simulink library "PCMULib"  (R2022b)
settings: Solver=ode45  StartTime=0.0  StopTime=10.0  RelTol=1e-3  EnableMultiTasking=on
undefined symbols (not defined in the file or in its folder): BreakpointData, BreakpointData1, BreakpointData2, BreakpointData_One_A, BreakpointData_Two_A, caaaa_dbi, caaaa_swi, cTmComprCtrl_n_i16SM4CmpHeatKiMax, cTmComprCtrl_n_i16SM4CmpHeatKiMin, cTmComprCtrl_n_i16SM4CmpHeatKpMax, cTmComprCtrl_n_i16SM4CmpHeatKpMin, cTmComprCtrl_Te_s32ErrCmpPIContinueHeatH, cTmComprCtrl_Te_s32ErrCmpPIContinueHeatL, cTmIn_n_ElacCmprReq_db, cTmIn_n_ElacCmprReq_sw, db, dbi, E2E_P01DataIDMode, E2E_P01ReceiverStatusType, EnumClass, iBit, initalValue, No_Runnable_Period, ObB_EidBsgStDerat_C, p_OVERRIDE_MASTER_SWITCH, SlDemoSign, sw, swi, SwitchOff_P, SwitchOn_P, Table, TableData_M, VCCTi33, VSysD_FidVehDerat1_C
libraries: simulink x22, CCMLib x11, simulink_need_slupdate x9, UXFD_Lib x7, canmsglib x2, PTCC_Lib x1, hdlsllib x1
(part 3 of 7)

== system PCMULib/CCM/Rate Limiter Resettable IC ==
  up : Inport  OutDataTypeStr=InputOutputDataType
  u : Inport  Port=2  OutDataTypeStr=InputOutputDataType
  IC : Inport  Port=3  OutDataTypeStr=InputOutputDataType
  T : Inport  Port=4  OutDataTypeStr=VCCTiSamplePerd
  lo : Inport  Port=5  OutDataTypeStr=InputOutputDataType
  R : Inport  Port=6  OutDataTypeStr=boolean
  Data Type Conversion{1..5} (5 alike) : DataTypeConversion  OutDataTypeStr=single  RndMeth=Floor
  Difference Inputs1 : Sum  Description=Add in CPU  DisableCoverage=on  Inputs=+-  OutDataTypeStr=single  SaturateOnIntegerOverflow=on
  Difference Inputs2 : Sum  Description=Add in CPU  OutDataTypeStr=single  SaturateOnIntegerOverflow=on
  FixPt Data Type Duplicate : DataTypeDuplicate  DisableCoverage=on  NumInputPorts=7
  Saturation Dynamic : simulink/Discontinuities/Saturation Dynamic  OutMin=[]  OutMax=[]  OutDataTypeStr=single  OutputDataTypeScalingMode=single  OutDataType=dataType  OutScaling=[]  DoSatur=on
  Switch : Switch  Criteria=u2 ~= 0  InputSameDT=off
  Unit Delay Resettable External IC boolean controlled : Subsystem  mask(Unit Delay Resettable External Initial Condition (boolean)){dt=single, UnitDelayInitCondition=0}
      mask prompts: dt "Data type in/out"; UnitDelayInitCondition "Internal unit delay block initial condition:"
      mask help:
      | This is the same block as the Simulink standard, except all fix point
      | data-types have been changed to booleans.
      | The internal unit delay block can often be kept as 0, unless the input/output signal is of ENUM type.
      | Made by Niklas Magnusson (nmagnus3).
      | NGCC
      mask Display: dpoly(1,[1 0],'z')
  dataType : DataTypeConversion  OutDataTypeStr=InputOutputDataType  RndMeth=Floor
  delta fall limit : Product  DisableCoverage=on  Inputs=**  OutDataTypeStr=single  SaturateOnIntegerOverflow=on
  delta rise limit : Product  DisableCoverage=on  Inputs=**  OutDataTypeStr=single  SaturateOnIntegerOverflow=on
  Y : Outport  OutDataTypeStr=InputOutputDataType  InitialOutput=0
  wires:
  Switch/1 -> dataType/1
  Data Type Conversion5/1 -> delta rise limit/2, delta fall limit/1
  R/1 -> Switch/2, Unit Delay Resettable External IC boolean controlled/2(R)
  IC/1 -> Data Type Conversion3/1
  Difference Inputs1/1 -> FixPt Data Type Duplicate/4, Saturation Dynamic/2
  u/1 -> Data Type Conversion2/1
  delta fall limit/1 -> FixPt Data Type Duplicate/3, Saturation Dynamic/3
  Saturation Dynamic/1 -> Difference Inputs2/1, FixPt Data Type Duplicate/7
  Unit Delay Resettable External IC boolean controlled/1(y) -> Difference Inputs2/2, Difference Inputs1/2, FixPt Data Type Duplicate/2
  Difference Inputs2/1 -> Switch/3, FixPt Data Type Duplicate/1, Unit Delay Resettable External IC boolean controlled/1(u)
  up/1 -> Data Type Conversion1/1
  delta rise limit/1 -> FixPt Data Type Duplicate/6, Saturation Dynamic/1
  lo/1 -> Data Type Conversion4/1
  T/1 -> Data Type Conversion5/1
  Data Type Conversion1/1 -> delta rise limit/1
  Data Type Conversion2/1 -> Difference Inputs1/1, FixPt Data Type Duplicate/5
  Data Type Conversion3/1 -> Switch/1, Unit Delay Resettable External IC boolean controlled/3(IC)
  Data Type Conversion4/1 -> delta fall limit/2
  dataType/1 -> Y/1

== system PCMULib/CCM/SR_latch ==
  Set : Inport  OutDataTypeStr=boolean
  Reset : Inport  Port=2  OutDataTypeStr=boolean
  Logical Operator : Logic  AllPortsSameDT=off  OutDataTypeStr=boolean
  Logical Operator1 : Logic  Operator=OR  AllPortsSameDT=off  OutDataTypeStr=boolean
  Logical Operator2 : Logic  Operator=NOT  AllPortsSameDT=off  OutDataTypeStr=boolean
  Unit Delay External IC : simulink_need_slupdate/Unit Delay External IC  tsamp=-1
  false : Constant  Value=false  OutDataTypeStr=boolean  SampleTime=-1
  SetState : Outport  OutDataTypeStr=boolean
  wires:
  Set/1 -> Logical Operator1/2
  false/1 -> Unit Delay External IC/2
  Unit Delay External IC/1 -> Logical Operator1/1
  Logical Operator2/1 -> Logical Operator/2
  Reset/1 -> Logical Operator2/1
  Logical Operator1/1 -> Logical Operator/1
  Logical Operator/1 -> Unit Delay External IC/1, SetState/1

== system PCMULib/CCM/SR_latch_NoRst ==
  Set : Inport  OutDataTypeStr=boolean
  Logical Operator1 : Logic  Operator=OR  AllPortsSameDT=off  OutDataTypeStr=boolean
  Unit Delay External IC : simulink_need_slupdate/Unit Delay External IC  tsamp=-1
  false : Constant  Value=false  OutDataTypeStr=boolean  SampleTime=-1
  SetState : Outport  OutDataTypeStr=boolean
  wires:
  Logical Operator1/1 -> SetState/1, Unit Delay External IC/1
  Unit Delay External IC/1 -> Logical Operator1/1
  false/1 -> Unit Delay External IC/2
  Set/1 -> Logical Operator1/2

== system PCMULib/CCM/Timer ==
  note: CounterRunning
  note: If timer is set to zero, use start/hold/reset-status as output.
      | This is to avoid TimerFinished to be set to true without even the timer has started.
  Start : Inport  OutDataTypeStr=boolean
  Reset : Inport  Port=2  OutDataTypeStr=boolean
  Time : Inport  Port=3  OutDataTypeStr=timeDataType
  Divide : Product  Inputs=*/  OutDataTypeStr=VCCUInt32  RndMeth=Round  SaturateOnIntegerOverflow=on
  IC : Constant  Value=0  OutDataTypeStr=VCCUInt32  SampleTime=-1
  Increment : Constant  OutDataTypeStr=VCCUInt32  SampleTime=-1
  Logical Operator : Logic  AllPortsSameDT=off  OutDataTypeStr=boolean
  Logical Operator2 : Logic  Operator=OR  AllPortsSameDT=off  OutDataTypeStr=boolean
  Logical Operator3 : Logic  Operator=NOT  AllPortsSameDT=off  OutDataTypeStr=boolean
  Relational Operator : RelationalOperator  OutDataTypeStr=boolean  InputSameDT=off
  Relational Operator1 : RelationalOperator  Operator=>  OutDataTypeStr=boolean  InputSameDT=off
  RunnablePeriod : Constant  Value=RunnablePeriod  OutDataTypeStr=VCCTiSamplePerd  SampleTime=-1
  StopCounter : Constant  Value=0  OutDataTypeStr=VCCUInt32  SampleTime=-1
  Sum : Sum  OutDataTypeStr=VCCUInt32  SaturateOnIntegerOverflow=on
  Switch : Switch  Criteria=u2 ~= 0  InputSameDT=off
  Switch1 : Switch  Criteria=u2 ~= 0  InputSameDT=off
  Unit Delay External IC : simulink_need_slupdate/Unit Delay External IC  tsamp=-1
  Unit Delay Resettable External IC1 : CCMLib/Unit Delay Resettable External IC  dataType=VCCUInt32
  ZeroTicks : Constant  Value=0  OutDataTypeStr=VCCUInt32  SampleTime=-1
  false : Constant  Value=false  OutDataTypeStr=boolean  SampleTime=-1
  TimerFinished : Outport  OutDataTypeStr=boolean
  wires:
  Logical Operator2/1 -> Logical Operator/1
  false/1 -> Unit Delay External IC/2
  Logical Operator/1 -> Switch/2, Unit Delay External IC/1, Switch1/3
  Start/1 -> Logical Operator2/2
  Unit Delay External IC/1 -> Logical Operator2/1
  Unit Delay Resettable External IC1/1 -> Sum/1, Relational Operator/1
  Switch/1 -> Sum/2
  Increment/1 -> Switch/1
  StopCounter/1 -> Switch/3
  RunnablePeriod/1 -> Divide/2
  ZeroTicks/1 -> Relational Operator1/2
  Relational Operator1/1 -> Switch1/2
  Relational Operator/1 -> Switch1/1
  Divide/1 -> Relational Operator/2, Relational Operator1/1
  Switch1/1 -> TimerFinished/1
  Logical Operator3/1 -> Logical Operator/2
  Reset/1 -> Logical Operator3/1, Unit Delay Resettable External IC1/3
  Time/1 -> Divide/1
  IC/1 -> Unit Delay Resettable External IC1/2
  Sum/1 -> Unit Delay Resettable External IC1/1

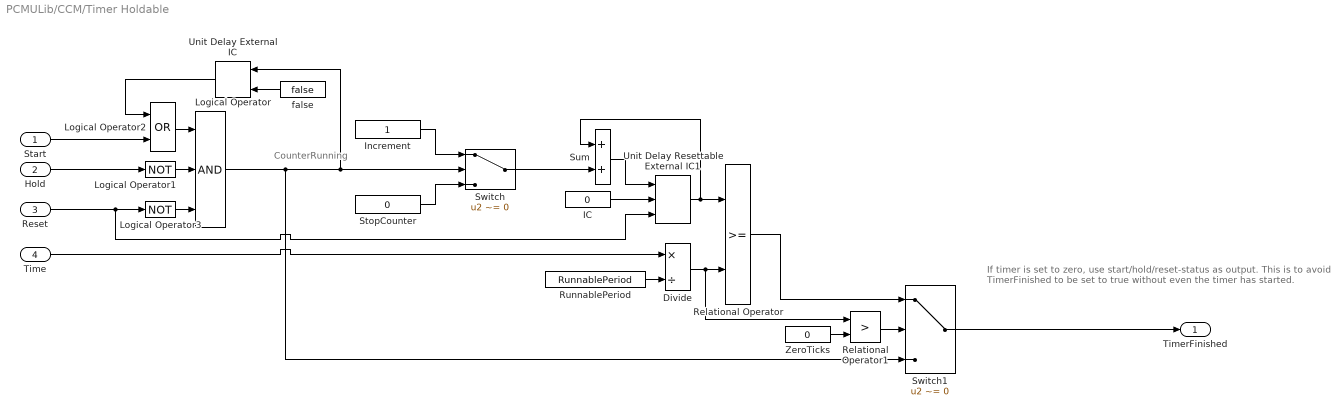
== system PCMULib/CCM/Timer Holdable ==
  note: If timer is set to zero, use start/hold/reset-status as output.
      | This is to avoid TimerFinished to be set to true without even the timer has started.
  note: CounterRunning
  Start : Inport  OutDataTypeStr=boolean
  Hold : Inport  Port=2  OutDataTypeStr=boolean
  Reset : Inport  Port=3  OutDataTypeStr=boolean
  Time : Inport  Port=4  OutDataTypeStr=timeDataType
  Divide : Product  Inputs=*/  OutDataTypeStr=VCCUInt32  RndMeth=Round  SaturateOnIntegerOverflow=on
  IC : Constant  Value=0  OutDataTypeStr=VCCUInt32  SampleTime=-1
  Increment : Constant  OutDataTypeStr=VCCUInt32  SampleTime=-1
  Logical Operator : Logic  Inputs=3  AllPortsSameDT=off  OutDataTypeStr=boolean
  Logical Operator1 : Logic  Operator=NOT  AllPortsSameDT=off  OutDataTypeStr=boolean
  Logical Operator2 : Logic  Operator=OR  AllPortsSameDT=off  OutDataTypeStr=boolean
  Logical Operator3 : Logic  Operator=NOT  AllPortsSameDT=off  OutDataTypeStr=boolean
  Relational Operator : RelationalOperator  OutDataTypeStr=boolean  InputSameDT=off
  Relational Operator1 : RelationalOperator  Operator=>  OutDataTypeStr=boolean  InputSameDT=off
  RunnablePeriod : Constant  Value=RunnablePeriod  OutDataTypeStr=VCCTiSamplePerd  SampleTime=-1
  StopCounter : Constant  Value=0  OutDataTypeStr=VCCUInt32  SampleTime=-1
  Sum : Sum  OutDataTypeStr=VCCUInt32  SaturateOnIntegerOverflow=on
  Switch : Switch  Criteria=u2 ~= 0  InputSameDT=off
  Switch1 : Switch  Criteria=u2 ~= 0  InputSameDT=off
  Unit Delay External IC : simulink_need_slupdate/Unit Delay External IC  tsamp=-1
  Unit Delay Resettable External IC1 : CCMLib/Unit Delay Resettable External IC  dataType=VCCUInt32
  ZeroTicks : Constant  Value=0  OutDataTypeStr=VCCUInt32  SampleTime=-1
  false : Constant  Value=false  OutDataTypeStr=boolean  SampleTime=-1
  TimerFinished : Outport  OutDataTypeStr=boolean
  wires:
  Sum/1 -> Unit Delay Resettable External IC1/1
  IC/1 -> Unit Delay Resettable External IC1/2
  Time/1 -> Divide/1
  Reset/1 -> Unit Delay Resettable External IC1/3, Logical Operator3/1
  Logical Operator3/1 -> Logical Operator/3
  Switch1/1 -> TimerFinished/1
  Divide/1 -> Relational Operator1/1, Relational Operator/2
  Relational Operator/1 -> Switch1/1
  Relational Operator1/1 -> Switch1/2
  ZeroTicks/1 -> Relational Operator1/2
  RunnablePeriod/1 -> Divide/2
  StopCounter/1 -> Switch/3
  Increment/1 -> Switch/1
  Switch/1 -> Sum/2
  Unit Delay Resettable External IC1/1 -> Relational Operator/1, Sum/1
  Unit Delay External IC/1 -> Logical Operator2/1
  Start/1 -> Logical Operator2/2
  Logical Operator/1 -> Switch1/3, Unit Delay External IC/1, Switch/2
  false/1 -> Unit Delay External IC/2
  Logical Operator2/1 -> Logical Operator/1
  Hold/1 -> Logical Operator1/1
  Logical Operator1/1 -> Logical Operator/2

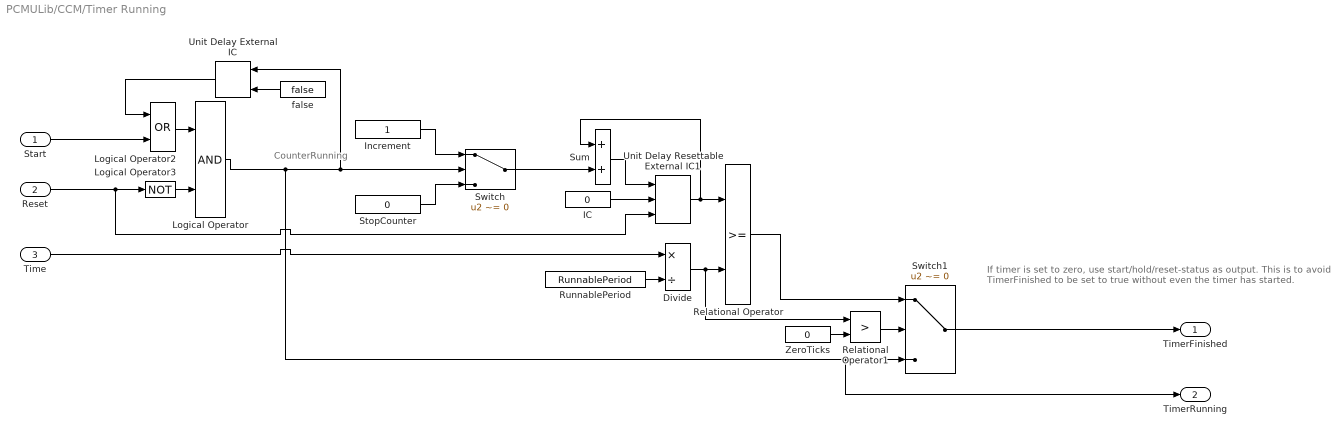
== system PCMULib/CCM/Timer Running ==
  note: If timer is set to zero, use start/hold/reset-status as output.
      | This is to avoid TimerFinished to be set to true without even the timer has started.
  note: CounterRunning
  Start : Inport  OutDataTypeStr=boolean
  Reset : Inport  Port=2  OutDataTypeStr=boolean
  Time : Inport  Port=3  OutDataTypeStr=timeDataType
  Divide : Product  Inputs=*/  OutDataTypeStr=VCCUInt32  RndMeth=Round  SaturateOnIntegerOverflow=on
  IC : Constant  Value=0  OutDataTypeStr=VCCUInt32  SampleTime=-1
  Increment : Constant  OutDataTypeStr=VCCUInt32  SampleTime=-1
  Logical Operator : Logic  AllPortsSameDT=off  OutDataTypeStr=boolean
  Logical Operator2 : Logic  Operator=OR  AllPortsSameDT=off  OutDataTypeStr=boolean
  Logical Operator3 : Logic  Operator=NOT  AllPortsSameDT=off  OutDataTypeStr=boolean
  Relational Operator : RelationalOperator  OutDataTypeStr=boolean  InputSameDT=off
  Relational Operator1 : RelationalOperator  Operator=>  OutDataTypeStr=boolean  InputSameDT=off
  RunnablePeriod : Constant  Value=RunnablePeriod  OutDataTypeStr=VCCTiSamplePerd  SampleTime=-1
  StopCounter : Constant  Value=0  OutDataTypeStr=VCCUInt32  SampleTime=-1
  Sum : Sum  OutDataTypeStr=VCCUInt32  SaturateOnIntegerOverflow=on
  Switch : Switch  Criteria=u2 ~= 0  InputSameDT=off
  Switch1 : Switch  Criteria=u2 ~= 0  InputSameDT=off
  Unit Delay External IC : simulink_need_slupdate/Unit Delay External IC  tsamp=-1
  Unit Delay Resettable External IC1 : CCMLib/Unit Delay Resettable External IC  dataType=VCCUInt32
  ZeroTicks : Constant  Value=0  OutDataTypeStr=VCCUInt32  SampleTime=-1
  false : Constant  Value=false  OutDataTypeStr=boolean  SampleTime=-1
  TimerFinished : Outport  OutDataTypeStr=boolean
  TimerRunning : Outport  Port=2  OutDataTypeStr=boolean
  wires:
  Sum/1 -> Unit Delay Resettable External IC1/1
  IC/1 -> Unit Delay Resettable External IC1/2
  Time/1 -> Divide/1
  Reset/1 -> Unit Delay Resettable External IC1/3, Logical Operator3/1
  Logical Operator3/1 -> Logical Operator/2
  Switch1/1 -> TimerFinished/1
  Divide/1 -> Relational Operator1/1, Relational Operator/2
  Relational Operator/1 -> Switch1/1
  Relational Operator1/1 -> Switch1/2
  ZeroTicks/1 -> Relational Operator1/2
  RunnablePeriod/1 -> Divide/2
  StopCounter/1 -> Switch/3
  Increment/1 -> Switch/1
  Switch/1 -> Sum/2
  Unit Delay Resettable External IC1/1 -> Sum/1, Relational Operator/1
  Unit Delay External IC/1 -> Logical Operator2/1
  Start/1 -> Logical Operator2/2
  Logical Operator/1 -> TimerRunning/1, Switch1/3, Unit Delay External IC/1, Switch/2
  false/1 -> Unit Delay External IC/2
  Logical Operator2/1 -> Logical Operator/1

== system PCMULib/CCM/Unit Delay External IC ==
  u : Inport  OutDataTypeStr=dataType
  IC : Inport  Port=2  OutDataTypeStr=dataType
  Constant : Constant  Value=true  OutDataTypeStr=boolean  SampleTime=-1
  Switch : Switch  Criteria=u2 ~= 0  InputSameDT=off
  Unit Delay : UnitDelay  InitialCondition=false  SampleTime=-1  HasFrameUpgradeWarning=on
      settings: AttributesFormatString=X0=%<X0>
  Unit Delay1 : UnitDelay  SampleTime=-1  HasFrameUpgradeWarning=on
      settings: AttributesFormatString=X0=%<X0>
  y : Outport  OutDataTypeStr=dataType
  wires:
  Switch/1 -> y/1
  IC/1 -> Switch/3
  u/1 -> Unit Delay1/1
  Unit Delay1/1 -> Switch/1
  Constant/1 -> Unit Delay/1
  Unit Delay/1 -> Switch/2

== system PCMULib/CCM/Unit Delay Resettable ==
  u : Inport  OutDataTypeStr=dataType
  R : Inport  Port=2  OutDataTypeStr=boolean
  Constant : Constant  Value=false  OutDataTypeStr=boolean  SampleTime=-1
  Logical Operator : Logic  Operator=OR  AllPortsSameDT=off  OutDataTypeStr=boolean
  Logical Operator1 : Logic  Operator=NOT  AllPortsSameDT=off  OutDataTypeStr=boolean
  Switch : Switch  Criteria=u2 ~= 0  InputSameDT=off
  Switch1 : Switch  Criteria=u2 ~= 0  InputSameDT=off
  Unit Delay : UnitDelay  InitialCondition=true  SampleTime=-1  HasFrameUpgradeWarning=on
      settings: AttributesFormatString=X0=%<X0>
  Unit Delay1 : UnitDelay  InitialCondition=initialCondition  SampleTime=-1  HasFrameUpgradeWarning=on
      settings: AttributesFormatString=X0=%<X0>
  initialCondition : Constant  Value=initialCondition  OutDataTypeStr=dataType  SampleTime=-1
  y : Outport  OutDataTypeStr=dataType
  wires:
  Constant/1 -> Unit Delay/1
  Switch/1 -> y/1
  Logical Operator/1 -> Switch/2
  Unit Delay/1 -> Logical Operator/2
  R/1 -> Logical Operator/1, Logical Operator1/1
  Logical Operator1/1 -> Switch1/2
  initialCondition/1 -> Switch1/3, Switch/1
  Switch1/1 -> Unit Delay1/1
  Unit Delay1/1 -> Switch/3
  u/1 -> Switch1/1

== system PCMULib/CCM/Unit Delay Resettable External IC ==
  u : Inport  OutDataTypeStr=dataType
  IC : Inport  Port=2  OutDataTypeStr=dataType
  R : Inport  Port=3  OutDataTypeStr=boolean
  Constant : Constant  Value=true  OutDataTypeStr=boolean  SampleTime=-1
  Logical Operator : Logic  Operator=NOT  AllPortsSameDT=off  OutDataTypeStr=boolean
  Logical Operator1 : Logic  AllPortsSameDT=off  OutDataTypeStr=boolean
  Switch : Switch  Criteria=u2 ~= 0  InputSameDT=off
  Switch1 : Switch  Criteria=u2 ~= 0  InputSameDT=off
  Unit Delay : UnitDelay  InitialCondition=false  SampleTime=-1  HasFrameUpgradeWarning=on
      settings: AttributesFormatString=X0=%<X0>
  Unit Delay1 : UnitDelay  SampleTime=-1  HasFrameUpgradeWarning=on
      settings: AttributesFormatString=X0=%<X0>
  y : Outport  OutDataTypeStr=dataType
  wires:
  Logical Operator1/1 -> Switch/2
  Unit Delay/1 -> Logical Operator1/1
  Switch1/1 -> Unit Delay1/1
  IC/1 -> Switch/3, Switch1/3
  u/1 -> Switch1/1
  R/1 -> Logical Operator/1
  Logical Operator/1 -> Logical Operator1/2, Switch1/2
  Constant/1 -> Unit Delay/1
  Unit Delay1/1 -> Switch/1
  Switch/1 -> y/1

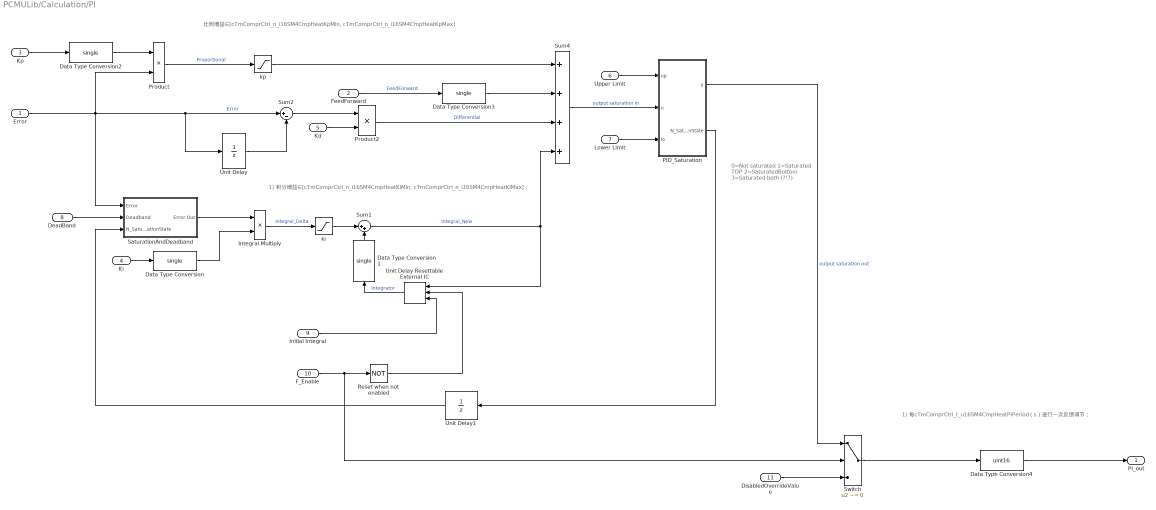
== system PCMULib/Calculation/PI ==
  note: 1) 积分增益∈[cTmComprCtrl_n_i16SM4CmpHeatKiMin, cTmComprCtrl_n_i16SM4CmpHeatKiMax]；
  note: 比例增益∈[cTmComprCtrl_n_i16SM4CmpHeatKpMin, cTmComprCtrl_n_i16SM4CmpHeatKpMax]
  note: 1) 每cTmComprCtrl_t_u16SM4CmpHeatPIPeriod（s）进行一次反馈调节；
  note: 0=Not saturated
      | 1=Saturated TOP
      | 2=SaturatedBottom
      | 3=Saturated both (?!?)
  Error : Inport  OutDataTypeStr=single
  FeedForward : Inport  Port=2  OutDataTypeStr=uint16
  Kp : Inport  Port=3  OutDataTypeStr=uint16
  Ki : Inport  Port=4  OutDataTypeStr=uint16
  Kd : Inport  Port=5  OutDataTypeStr=single
  Upper Limit : Inport  Port=6  OutDataTypeStr=single
  Lower Limit : Inport  Port=7  OutDataTypeStr=single
  DeadBand : Inport  Port=8  OutDataTypeStr=single
  Initial Integral : Inport  Port=9  OutDataTypeStr=single
  F_Enable : Inport  Port=10  OutDataTypeStr=boolean
  DisabledOverrideValue : Inport  Port=11  OutDataTypeStr=single
  Data Type Conversion{,1..3} (4 alike) : DataTypeConversion  OutDataTypeStr=single  SaturateOnIntegerOverflow=off  RndMeth=Floor
  Data Type Conversion4 : DataTypeConversion  OutDataTypeStr=uint16  SaturateOnIntegerOverflow=off  RndMeth=Floor
  Integral Multiply : Product  OutDataTypeStr=single  RndMeth=Zero  SaturateOnIntegerOverflow=on
  PID_Saturation : Subsystem  mask(Saturation Dynamic){OutMin=[], OutMax=[], OutDataTypeStr=Inherit: Same as second input, OutputDataTypeScalingMode=Same as second input, OutDataType=FloatBit1, OutScaling=[], LockScale=off, RndMeth=Nearest, DoSatur=on}
      mask prompts: OutMin "Output minimum:"; OutMax "Output maximum:"; OutDataTypeStr "Output data type:"; OutputDataTypeScalingMode "Output data type mode:"; OutDataType "Output data type (e.g. fixdt(1, 16), fixdt('single')):"; OutScaling "Output scaling (Slope, e.g. 2^-9 or [Slope Bias], e.g. [1.25 3]):"; LockScale "Lock output data type setting against changes by the fixed-point tools"; RndMeth "Integer rounding mode:"; DoSatur "Saturate on integer overflow"
      mask help: Bound the range of the second input by using the first input (upper limit) and the third input (lower limit).
      mask init:
      | blkH = gcbh;
      | blkName = getfullname(blkH);
      | 
      | switch_blks = {'Switch','Switch2'}; 
      | for i = 1:length(switch_blks)
      |   set_param([blkName,'/',switch_blks{i}], ...
      |       'RndMeth', RndMeth, ...
      | 	  'DoSatur', DoSatur);
      | end
      | 
      | propBlk = [blkName, '/Data Type Propagation'];
      | 
      | if strcmp(OutputDataTypeScalingMode, 'Same as second input')
      |     set_param(propBlk, 'PropDataTypeMode', 'Inherit via propagation rule', ...
      |                        'PropScalingMode',  'Inherit via propagation rule');
      | else
      |     scaling = OutScaling;
      |     switch OutputDataTypeScalingMode
      |       case 'double'
      |         dataType = 'fixdt(''double'')';
      |       case 'single'
      |         dataType = 'fixdt(''single'')';
      |       case 'int8'
      |         dataType = 'fixdt(1,8,0)';
      |       case 'uint8'
      |         dataType = 'fixdt(0,8,0)';
      |       case 'int16'
      |         dataType = 'fixdt(1,16,0)';
      |       case 'uint16'
      |         dataType = 'fixdt(0,16,0)';
      |       case 'int32'
      |         dataType = 'fixdt(1,32,0)';
      |       case 'uint32'
      |         dataType = 'fixdt(0,32,0)';
      |       case 'Specify via dialog'
      |         dataType = OutDataType;
      |     end
      |     
      |     set_param(propBlk, 'PropDataTypeMode', 'Specify via dialog', ...
      |                        'PropScalingMode',  'Specify via dialog', ...
      |                        'PropDataType',     dataType, ...
      |                        'PropScaling',      scaling);
      | end
      mask Callback OutDataTypeStr: fixptdialog(gcbh)
      mask TypeOptions OutputDataTypeScalingMode: double | single | int8 | uint8 | int16 | uint16 | int32 | uint32 | Specify via dialog | Same as second input
      mask Callback OutputDataTypeScalingMode: fixptdialog(gcbh)
      mask Callback OutDataType: fixptdialog(gcbh)
      mask TypeOptions RndMeth: Ceiling | Convergent | Floor | Nearest | Round | Simplest | Zero
      mask Display: plot([0.15 0.85],[.5 .5],[.5 .5],[0.05 0.95],0.15+0.7*[0 .25 .75 1],0.05+0.9*[.25 .25 .75 .75]);
  Product : Product  OutDataTypeStr=single  RndMeth=Zero
  Product2 : Product  OutDataTypeStr=single  RndMeth=Zero  SaturateOnIntegerOverflow=on
  Reset when not enabled : Logic  Operator=NOT  Inputs=1  AllPortsSameDT=off  OutDataTypeStr=boolean
  SaturationAndDeadband : Subsystem
  Sum1 : Sum  Inputs=|++  InputSameDT=on  AccumDataTypeStr=single  OutDataTypeStr=single  SaturateOnIntegerOverflow=on
  Sum2 : Sum  Inputs=|+-  SaturateOnIntegerOverflow=on
  Sum4 : Sum  Inputs=++++  RndMeth=Nearest  SaturateOnIntegerOverflow=on
  Switch : Switch  Criteria=u2 ~= 0  SaturateOnIntegerOverflow=off  InputSameDT=off
  Unit Delay : UnitDelay  SampleTime=-1  HasFrameUpgradeWarning=on
  Unit Delay Resettable External IC : simulink_need_slupdate/Unit Delay Resettable External IC  tsamp=-1
  Unit Delay1 : UnitDelay  SampleTime=-1  HasFrameUpgradeWarning=on
  ki : Saturate  UpperLimit=cTmComprCtrl_n_i16SM4CmpHeatKiMax  LowerLimit=cTmComprCtrl_n_i16SM4CmpHeatKiMin
  kp : Saturate  UpperLimit=cTmComprCtrl_n_i16SM4CmpHeatKpMax  LowerLimit=cTmComprCtrl_n_i16SM4CmpHeatKpMin
  PI_out : Outport  OutDataTypeStr=uint16  VectorParamsAs1DForOutWhenUnconnected=off
  wires:
  Product2/1 -> Sum4/3  "Differential"
  Sum1/1 -> Sum4/4, Unit Delay Resettable External IC/1  "Integral_New"
  Upper Limit/1 -> PID_Saturation/1(up)
  DeadBand/1 -> SaturationAndDeadband/2(Deadband)
  Unit Delay/1 -> Sum2/2
  Kd/1 -> Product2/2
  DisabledOverrideValue/1 -> Switch/3
  Error/1 -> SaturationAndDeadband/1(Error), Product/2, Sum2/1, Unit Delay/1  "Error"
  Sum2/1 -> Product2/1
  Unit Delay Resettable External IC/1 -> Data Type Conversion1/1  "Integrator"
  Kp/1 -> Data Type Conversion2/1
  PID_Saturation/1(y) -> Switch/1  "output saturation out"
  Reset when not enabled/1 -> Unit Delay Resettable External IC/2
  Initial Integral/1 -> Unit Delay Resettable External IC/3
  Lower Limit/1 -> PID_Saturation/3(lo)
  SaturationAndDeadband/1(Error Out) -> Integral Multiply/1
  Sum4/1 -> PID_Saturation/2(u)  "output saturation in"
  FeedForward/1 -> Data Type Conversion3/1  "FeedForward"
  F_Enable/1 -> Reset when not enabled/1, Switch/2
  Unit Delay1/1 -> SaturationAndDeadband/3(N_SaturationState)
  Product/1 -> kp/1  "Proportional"
  Integral Multiply/1 -> ki/1  "Integral_Delta"
  PID_Saturation/2(N_SaturationState) -> Unit Delay1/1
  Ki/1 -> Data Type Conversion/1
  Data Type Conversion1/1 -> Sum1/2
  kp/1 -> Sum4/1
  ki/1 -> Sum1/1
  Switch/1 -> Data Type Conversion4/1
  Data Type Conversion/1 -> Integral Multiply/2
  Data Type Conversion2/1 -> Product/1
  Data Type Conversion3/1 -> Sum4/2
  Data Type Conversion4/1 -> PI_out/1

== system PCMULib/Calculation/interpolation ==
  note: 外循环比例
  note: 内循环比例
  rate : Inport
  internal : Inport  Port=2
  external : Inport  Port=3
  Add1 : Sum  Inputs=-+
  Add2 : Sum
  Constant4 : Constant  OutDataTypeStr=single
  Constant5 : Constant  Value=100  OutDataTypeStr=single
  Data Type Conversion : DataTypeConversion  OutDataTypeStr=uint16  SaturateOnIntegerOverflow=off  RndMeth=Floor
  Product : Product
  Product1 : Product
  Product2 : Product  Inputs=*/
  rst : Outport
  wires:
  external/1 -> Product1/2
  Product1/1 -> Add2/2
  Add2/1 -> Data Type Conversion/1
  rate/1 -> Product2/1
  Constant4/1 -> Add1/2
  Product/1 -> Add2/1
  internal/1 -> Product/1
  Add1/1 -> Product1/1
  Constant5/1 -> Product2/2
  Product2/1 -> Product/2, Add1/1
  Data Type Conversion/1 -> rst/1

== system PCMULib/Custom/CAN ==
  note: CAN
  CAN Pack : canmsglib/CAN Pack  MsgList=(none)  MsgName=CAN Msg  MsgIDType=Standard (11-bit identifier)  MsgIdentifier=0  MsgLength=8  Remote=off  ApplyMinMax=off  BusOutput=off  SignalInfo={}
      settings: DataFormat=raw data
  CAN Unpack : canmsglib/CAN Unpack  MsgList=(none)  MsgName=CAN Msg  MsgIDType=Standard (11-bit identifier)  MsgIdentifier=0  MsgLength=8  SignalInfo={}  IDPort=off  TimestampPort=off  ErrorPort=off  RemotePort=off  LengthPort=off  StatusPort=off  ApplyMinMax=off
      settings: DataFormat=raw data
  CAN_Receive : Subsystem  mask(CAN Message Receive( GLib TM )){}
      mask help:
      | Input： DataType CAN_Message Signal and handle
      | Output：If Received success , Return Value is 1
      mask Display:
      | port_label('input',1,'Message')
      | port_label('input',2,'Handle')
      | port_label('output',1,'ReturnValue')
      | disp('ACTION_CANBSW_RecMsg_S')
  CAN_Transmit : Subsystem  mask(CAN Message Transmit( GLib TM )){}
      mask help:
      | Input： DataType CAN_Message Signal and handle
      | Output：If Transmited success , Return Value is 1
      mask Display:
      | port_label('input',1,'Message')
      | port_label('input',2,'Handle')
      | port_label('output',1,'ReturnValue')
      | disp('ACTION_CANBSW_SndMsg_S')
  CanHex2Signed : Subsystem  mask(CAN signal Hex2Signed){BitLengthValue=32, FactorValue=0.001, OffsetValue=0}
      mask prompts: BitLengthValue "CAN Signal Bit Length（0<u<=32bit）"; FactorValue "Factor"; OffsetValue "Offset"
      mask help: convert the hex to signed value, please specified bit length of varible in CAN matrix, the maximum bit length in CAN matrixa may be 32bit; Also, please specified the factor and offset, then execute Phy=hex*factor+offset.
      mask init:
      | % The mask parameter returns the one-based index of the selection
      | FactorValue;
      | OffsetValue;
      | BitLengthValue;
      | % To obtain the string corresponding to the selection, use get_param
      | blk = gcb;
      | FactorString = get_param(blk,'FactorValue');
      | OffsetString = get_param(blk,'OffsetValue');
      | BitSzieString = get_param(blk,'BitLengthValue');
      | 
      |     % Convert the string into a single to use the value under the mask
      |     BitLength = single(str2num(BitSzieString)); 
      |     Factor=single(str2num(FactorString)); 
      |     Offset=single(str2num(OffsetString));
      mask Display:
      | fprintf('CAN signal convert\nBitLength: %d\nFactor: %2.4f\nOffset: %2.4f',...
      |     BitLengthValue,FactorValue,OffsetValue);
  Get_MsgLength : Subsystem  mask(Get CAN Message Length( GLib TM )){}
      mask help:
      | Input： DataType CAN_Message Signal
      | Output：CAN Message Length
      mask Display:
      | port_label('input',1,'Message')
      | port_label('output',1,'Length')
      | disp('Msg_Length_S')
  xbackground1 : Subsystem
      mask Display: disp(' ')

== system PCMULib/Custom/Diagnose ==
  note: Diagnose
  Dem_SetEventStatus : Subsystem  mask(SL Blockset Dem_SetEventStatus){EventID=ObB_EidBsgStDerat_C}
      mask prompts: EventID "Dem Event ID"
      mask help:
      | Interface block to call Dem_SetEventStatus.
      | The output of the block can be captured by using Dem_SetEventStatus blocks with the same EventID.
      mask TypeOptions EventID: DEM_EventID/Value
      mask Display:
      | id = get_param(gcb,'EventID');
      | text(0.55,0.9,sprintf('Dem_SetEventStatus\nEventID: %s', id),...
      |     'horizontalAlignment','center',...
      |     'verticalAlignment', 'top');
      | 
      | 
      | port_label('input',1,'EveSt');
      | port_label('input',2,'bEna');
  Fim_GetFunctionPermission : Subsystem  mask(SL Blockset Fim_GetFunctionPermission){FunctionID=VSysD_FidVehDerat1_C}
      mask prompts: FunctionID "FIM FunctionID"
      mask help:
      | Interface block to call Fim_GetFunctionPermission.
      | The output of the block can be stimulated by using Fim_GetFunctionPermission_Stimuli blocks with the same FunctionID.
      mask TypeOptions FunctionID: FIM_EventID/Value
      mask Display:
      | id = get_param(gcb,'FunctionID');
      | text(0.45,0.9,sprintf('Fim_GetFunctionPermission\nFunctionID: %s', id),...
      |     'horizontalAlignment','center',...
      |     'verticalAlignment', 'top');
      | 
      | port_label('output',1,'bEna');
  xbackground1 : Subsystem
      mask Display: disp(' ')

== system PCMULib/Custom/PIN ==
  note: HW PIN
  PIN ADC : Subsystem  mask(PIN ADC){g_functionName=Sws_Io_Adc_Get_xxx, g_getValue=2}
      mask prompts: g_functionName "应用层接口函数"; g_getValue "测试输出返回值"
      mask help:
      | This block is for ASW to get Hardware's  ADC PIN Value
      | Function: uint16 Sws_Io_Adc_Get_xxx(void)
      mask Display: text(0.08,0.67,'Get Pin Analog Input','horizontalAlignment', 'left', 'verticalAlignment', 'top');
  PIN DI : Subsystem  mask(PIN DI){g_functionName=Sws_Io_Dio_Get_xxx, g_getValue=1}
      mask prompts: g_functionName "应用层接口函数"; g_getValue "测试输出返回值"
      mask help:
      | This block is for ASW to get Hardware's  DI PIN Value
      | Function: boolean Sws_Io_Dio_Get_xxx()
      mask Display: text(0.08,0.67,'Get Pin Digital Input','horizontalAlignment', 'left', 'verticalAlignment', 'top');
  PIN DO : Subsystem  mask(PIN DO){g_functionName=Sws_Io_Dio_Set_O_S_xxx}
      mask prompts: g_functionName "应用层接口函数"
      mask help:
      | This block is for ASW to set Hardware's  DO PIN Value
      | Function:  void Sws_Io_Dio_Set_O_S_xxx(boolean stSignal_b)
      mask Display: text(0.08,0.67,'Set Pin Digital Output','horizontalAlignment', 'left', 'verticalAlignment', 'top');
  PIN DO1 : Subsystem  mask(PIN PWMOUT){g_functionName=Sws_Io_PWM_Set_O_S_xxx}
      mask prompts: g_functionName "应用层接口函数"
      mask help:
      | This block is for ASW to set Hardware's  PWM PIN Value
      | Function:  void Sws_Io_PWM_Set_O_S_xxx(sint16 Duty_s16,uint32 Period_u32)
      mask Display: text(0.08,0.67,'Set Pin PWM Output','horizontalAlignment', 'left', 'verticalAlignment', 'top');
  PIN ICU : Subsystem  mask(PIN ICU){g_functionName=Sws_Io_Icu_GetPeriod_xxx, g_getValue=50}
      mask prompts: g_functionName "应用层接口函数"; g_getValue "测试输出返回值"
      mask help:
      | This block is for ASW to get Hardware's  ICU PIN Value
      | Function:  Sws_Io_Icu_GetDutyCyclexxx(void)
      mask Display: text(0.08,0.67,'Get Pin ICU Input','horizontalAlignment', 'left', 'verticalAlignment', 'top');
  xbackground1 : Subsystem
      mask Display: disp(' ')

== system PCMULib/Interface/Indebug ==
  In1 : Inport
  DBI : Constant  Value=DBI
  SWI : Constant  Value=SWI
  Switch : Switch  Criteria=u2 ~= 0  SaturateOnIntegerOverflow=off  InputSameDT=off
  Out : Outport
  wires:
  Switch/1 -> Out/1
  SWI/1 -> Switch/2
  DBI/1 -> Switch/1
  In1/1 -> Switch/3

== system PCMULib/Interface/IndebugRvs ==
  In1 : Inport
  DBI : Constant  Value=DBI
  SWI : Constant  Value=SWI
  Switch : Switch  Criteria=u2 ~= 0  SaturateOnIntegerOverflow=off  InputSameDT=off
  Out : Outport
  wires:
  Switch/1 -> Out/1
  SWI/1 -> Switch/2
  DBI/1 -> Switch/1
  In1/1 -> Switch/3

== system PCMULib/Interface/Outdebug ==
  In1 : Inport
  DBI : Constant  Value=DBI
  SWI : Constant  Value=SWI
  Switch : Switch  Criteria=u2 ~= 0  SaturateOnIntegerOverflow=off  InputSameDT=off
  Out : Outport
  wires:
  Switch/1 -> Out/1
  SWI/1 -> Switch/2
  DBI/1 -> Switch/1
  In1/1 -> Switch/3

== system PCMULib/Interface/OutdebugRvs ==
  In1 : Inport
  DBI : Constant  Value=DBI
  SWI : Constant  Value=SWI
  Switch : Switch  Criteria=u2 ~= 0  SaturateOnIntegerOverflow=off  InputSameDT=off
  Out : Outport
  wires:
  In1/1 -> Switch/3
  DBI/1 -> Switch/1
  SWI/1 -> Switch/2
  Switch/1 -> Out/1

== system PCMULib/Standard/Bit Operation ==
  Bit Clear : simulink/Logic and Bit Operations/Bit Clear  iBit=0
  Bit Set : simulink/Logic and Bit Operations/Bit Set  iBit=0
  Bit Shift : hdlsllib/Logic and Bit Operations/Bit Shift  mode=Shift Left Logical  N=0
  Bitwise OR : simulink/Logic and Bit Operations/Bitwise Operator  logicop=OR  UseBitMask=off  BitMask=2.^iBit  BitMaskRealWorld=Stored Integer
  Bitwise Operator : simulink/Logic and Bit Operations/Bitwise Operator  logicop=AND  UseBitMask=on  BitMask=bin2dec('11011001')  BitMaskRealWorld=Stored Integer
  GetBitFnc : Subsystem  mask(Bit Get){GetBitPar=2, U8Par=uint32, BitMinPar=0, BitMaxPar=31}
      mask prompts: GetBitPar "GetBit"; U8Par "DataTypeSelect"; BitMinPar "BitMin"; BitMaxPar "BitMax"
      mask help: Input bit value, then select the bit position you want
      settings: CopyFcn=set_param(gcb, 'LinkStatus', 'none');
      mask Callback GetBitPar:
      | if isequal(get_param(gcb,'U8Par'),'uint8')
      |     set_param(gcb,'BitMinPar','0');
      |     set_param(gcb,'BitMaxPar','7');
      |     if str2double(get_param(gcb,'GetBitPar')) > 7
      |         set_param(gcb,'GetBitPar','7');
      |     elseif str2double(get_param(gcb,'GetBitPar')) < 0
      |         set_param(gcb,'GetBitPar','0');
      |     else
      |         set_param(gcb,'GetBitPar',num2str(uint8(str2double(get_param(gcb,'GetBitPar')))));
      |     end
      | elseif isequal(get_param(gcb,'U8Par'),'uint16')
      |     set_param(gcb,'BitMinPar','0');
      |     set_param(gcb,'BitMaxPar','15');
      |     if str2double(get_param(gcb,'GetBitPar')) > 15
      |         set_param(gcb,'GetBitPar','15');
      |     elseif str2double(get_param(gcb,'GetBitPar')) < 0
      |         set_param(gcb,'GetBitPar','0');
      |     else
      |         set_param(gcb,'GetBitPar',num2str(uint16(str2double(get_param(gcb,'GetBitPar')))));
      |     end
      | else
      |     set_param(gcb,'BitMinPar','0');
      |     set_param(gcb,'BitMaxPar','31');
      |     if str2double(get_param(gcb,'GetBitPar')) > 31
      |         set_param(gcb,'GetBitPar','31');
      |     elseif str2double(get_param(gcb,'GetBitPar')) < 0
      |         set_param(gcb,'GetBitPar','0');
      |     else
      |         set_param(gcb,'GetBitPar',num2str(uint32(str2double(get_param(gcb,'GetBitPar')))));
      |     end
      | end
      | set_param([gcb '/Getbit_n'],'value',['uint8(' get_param(gcb,'GetBitPar') ')']);
      mask TypeOptions U8Par: uint8 | uint16 | uint32
      mask Callback U8Par:
      | if isequal(get_param(gcb,'U8Par'),'uint8')
      |     set_param(gcb,'BitMinPar','0');
      |     set_param(gcb,'BitMaxPar','7');
      |     if str2double(get_param(gcb,'GetBitPar')) > 7
      |         set_param(gcb,'GetBitPar','7');
      |     elseif str2double(get_param(gcb,'GetBitPar')) < 0
      |         set_param(gcb,'GetBitPar','0');
      |     end
      | %     set_param([gcb '/BitWise'],'BitMask',['bin2dec(' '''' '11111111' '''' ')']);
      |     set_param([gcb '/Min'],'value','uint8(0)');
      |     set_param([gcb '/Max'],'value','uint8(7)');
      |     set_param([gcb '/BitVal'],'OutDataTypeStr','uint8');
      | elseif isequal(get_param(gcb,'U8Par'),'uint16')
      |     set_param(gcb,'BitMinPar','0');
      |     set_param(gcb,'BitMaxPar','15');
      |     if str2double(get_param(gcb,'GetBitPar')) > 15
      |         set_param(gcb,'GetBitPar','15');
      |     elseif str2double(get_param(gcb,'GetBitPar')) < 0
      |         set_param(gcb,'GetBitPar','0');
      |     end
      | %     set_param([gcb '/BitWise'],'BitMask',['bin2dec(' '''' '1111111111111111' '''' ')']);
      |     set_param([gcb '/Min'],'value','uint8(0)');
      |     set_param([gcb '/Max'],'value','uint8(15)');
      |     set_param([gcb '/BitVal'],'OutDataTypeStr','uint16');
      | else
      |     set_param(gcb,'BitMinPar','0');
      |     set_param(gcb,'BitMaxPar','31');
      |     if str2double(get_param(gcb,'GetBitPar')) > 31
      |         set_param(gcb,'GetBitPar','31');
      |     elseif str2double(get_param(gcb,'GetBitPar')) < 0
      |         set_param(gcb,'GetBitPar','0');
      |     end
      | %     set_param([gcb '/BitWise'],'BitMask',['bin2dec(' '''' '11111111111111111111111111111111' '''' ')']);
      |     set_param([gcb '/Min'],'value','uint8(0)');
      |     set_param([gcb '/Max'],'value','uint8(31)');
      |     set_param([gcb '/BitVal'],'OutDataTypeStr','uint32');
      | end
      mask Display:
      | % disp(dispStr)
      | % id = get_param(gcb,'GetBitPar');
      | % text(0.55,0.9,sprintf('Getbit_Uint8\n', id),...
      | %     'horizontalAlignment','center',...
      | %     'verticalAlignment', 'top');
      | disp([GetBitPar]);
      | port_label('input', 1, 'BitVal_B');
      | port_label('output', 1, 'Val');
  SetBitFnc : Subsystem  mask(Bit Set){SetBitPar=5, U8Par=uint32, BitMinPar=0, BitMaxPar=31}
      mask prompts: SetBitPar "SetBit"; U8Par "DataTypeSelect"; BitMinPar "BitMin"; BitMaxPar "BitMax"
      mask help: Input bit value, then select the bit position you want
      mask Callback SetBitPar:
      | if isequal(get_param(gcb,'U8Par'),'uint8')
      |     set_param(gcb,'BitMinPar','0');
      |     set_param(gcb,'BitMaxPar','7');
      |     if str2double(get_param(gcb,'SetBitPar')) > 7
      |         set_param(gcb,'SetBitPar','7');
      |     elseif str2double(get_param(gcb,'SetBitPar')) < 0
      |         set_param(gcb,'SetBitPar','0');
      |     else
      |         set_param(gcb,'SetBitPar',num2str(uint8(str2double(get_param(gcb,'SetBitPar')))));
      |     end
      | elseif isequal(get_param(gcb,'U8Par'),'uint16')
      |     set_param(gcb,'BitMinPar','0');
      |     set_param(gcb,'BitMaxPar','15');
      |     if str2double(get_param(gcb,'SetBitPar')) > 15
      |         set_param(gcb,'SetBitPar','15');
      |     elseif str2double(get_param(gcb,'SetBitPar')) < 0
      |         set_param(gcb,'SetBitPar','0');
      |     else
      |         set_param(gcb,'SetBitPar',num2str(uint16(str2double(get_param(gcb,'SetBitPar')))));
      |     end
      | else
      |     set_param(gcb,'BitMinPar','0');
      |     set_param(gcb,'BitMaxPar','31');
      |     if str2double(get_param(gcb,'SetBitPar')) > 31
      |         set_param(gcb,'SetBitPar','31');
      |     elseif str2double(get_param(gcb,'SetBitPar')) < 0
      |         set_param(gcb,'SetBitPar','0');
      |     else
      |         set_param(gcb,'SetBitPar',num2str(uint32(str2double(get_param(gcb,'SetBitPar')))));
      |     end
      | end
      | set_param([gcb '/Setbit_n'],'value',['uint8(' get_param(gcb,'SetBitPar') ')']);
      mask TypeOptions U8Par: uint8 | uint16 | uint32
      mask Callback U8Par:
      | if isequal(get_param(gcb,'U8Par'),'uint8')
      |     set_param(gcb,'BitMinPar','0');
      |     set_param(gcb,'BitMaxPar','7');
      |     if str2double(get_param(gcb,'SetBitPar')) > 7
      |         set_param(gcb,'SetBitPar','7');
      |     elseif str2double(get_param(gcb,'SetBitPar')) < 0
      |         set_param(gcb,'SetBitPar','0');
      |     end
      |     set_param([gcb '/BitWise'],'BitMask',['bin2dec(' '''' '11111111' '''' ')']);
      |     set_param([gcb '/Min'],'value','uint8(0)');
      |     set_param([gcb '/Max'],'value','uint8(7)');
      |     set_param([gcb '/Product'],'OutDataTypeStr','uint8');
      | elseif isequal(get_param(gcb,'U8Par'),'uint16')
      |     set_param(gcb,'BitMinPar','0');
      |     set_param(gcb,'BitMaxPar','15');
      |     if str2double(get_param(gcb,'SetBitPar')) > 15
      |         set_param(gcb,'SetBitPar','15');
      |     elseif str2double(get_param(gcb,'SetBitPar')) < 0
      |         set_param(gcb,'SetBitPar','0');
      |     end
      |     set_param([gcb '/BitWise'],'BitMask',['bin2dec(' '''' '1111111111111111' '''' ')']);
      |     set_param([gcb '/Min'],'value','uint8(0)');
      |     set_param([gcb '/Max'],'value','uint8(15)');
      |     set_param([gcb '/Product'],'OutDataTypeStr','uint16');
      | else
      |     set_param(gcb,'BitMinPar','0');
      |     set_param(gcb,'BitMaxPar','31');
      |     if str2double(get_param(gcb,'SetBitPar')) > 31
      |         set_param(gcb,'SetBitPar','31');
      |     elseif str2double(get_param(gcb,'SetBitPar')) < 0
      |         set_param(gcb,'SetBitPar','0');
      |     end
      |     set_param([gcb '/BitWise'],'BitMask',['bin2dec(' '''' '11111111111111111111111111111111' '''' ')']);
      |     set_param([gcb '/Min'],'value','uint8(0)');
      |     set_param([gcb '/Max'],'value','uint8(31)');
      |     set_param([gcb '/Product'],'OutDataTypeStr','uint32');
      | end
      mask Display:
      | disp([SetBitPar]);
      | port_label('input', 1, 'BitVal_B');
      | port_label('output', 1, 'Val');
  Shift Arithmetic : ArithShift  BitShiftNumber=8
      settings: CopyFcn=set_param(gcbh,'ShowName','off');
  xbackground4 : UXFD_Lib/xbackground4  SystemSampleTime=-1  VariantActivationTime=update diagram  Latency=0  AutoFrameSizeCalculation=off
